simulink model "Trigonometry"  (R2017b)
settings: Solver=FixedStepAuto  StartTime=0.0  StopTime=10.0  FixedStep=0.1  RelTol=1e-3  EnableMultiTasking=on
model workspace (MAT data in the model file):
  lustrec_slx_eps = 0.001
settings Model: Creator=ktrinh  LastModifiedBy=hbourbou
settings DataIOCC: SaveFormat=StructureWithTime
settings OptimizationCC: LifeSpan=inf
settings DebuggingCC: SFUnexpectedBacktrackingDiag=warning  SFNoUnconditionalDefaultTransitionDiag=warning  SFExecutionAtInitializationDiag=none
settings HardwareCC: ProdBitPerSizeT=32  ProdBitPerPtrDiffT=32  ProdWordSize=32  ProdHWDeviceType=Specified
settings CodeAppCC: StateflowObjectComments=on
settings GRTTargetCC: TargetLangStandard=C89/C90 (ANSI)  GeneratePreprocessorConditionals=Disable all
settings ConfigComp: CovMetricSettings=dw  CovHtmlReporting=on  CovSaveCumulativeToWorkspaceVar=on  CovSaveSingleToWorkspaceVar=on  CovExternalEMLEnable=off

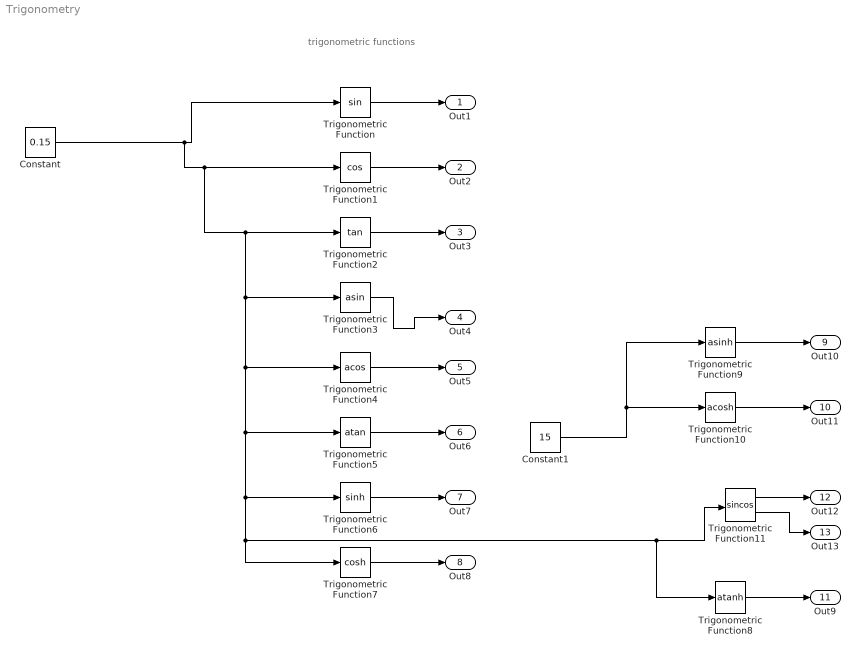
== system Trigonometry ==
  note: trigonometric functions
  Constant : Constant  Value=0.15
  Constant1 : Constant  Value=15
  Trigonometric Function : Trigonometry  ApproximationMethod=CORDIC
  Trigonometric Function1 : Trigonometry  Operator=cos  ApproximationMethod=CORDIC
  Trigonometric Function10 : Trigonometry  Operator=acosh  ApproximationMethod=CORDIC
  Trigonometric Function11 : Trigonometry  Operator=sincos  ApproximationMethod=CORDIC
  Trigonometric Function2 : Trigonometry  Operator=tan  ApproximationMethod=CORDIC
  Trigonometric Function3 : Trigonometry  Operator=asin  ApproximationMethod=CORDIC
  Trigonometric Function4 : Trigonometry  Operator=acos  ApproximationMethod=CORDIC
  Trigonometric Function5 : Trigonometry  Operator=atan  ApproximationMethod=CORDIC
  Trigonometric Function6 : Trigonometry  Operator=sinh  ApproximationMethod=CORDIC
  Trigonometric Function7 : Trigonometry  Operator=cosh  ApproximationMethod=CORDIC
  Trigonometric Function8 : Trigonometry  Operator=atanh  ApproximationMethod=CORDIC
  Trigonometric Function9 : Trigonometry  Operator=asinh  ApproximationMethod=CORDIC
  Out1 : Outport
  Out2 : Outport  Port=2
  Out3 : Outport  Port=3
  Out4 : Outport  Port=4
  Out5 : Outport  Port=5
  Out6 : Outport  Port=6
  Out7 : Outport  Port=7
  Out8 : Outport  Port=8
  Out10 : Outport  Port=9
  Out11 : Outport  Port=10
  Out9 : Outport  Port=11
  Out12 : Outport  Port=12
  Out13 : Outport  Port=13
  wires:
  Trigonometric Function/1 -> Out1/1
  Trigonometric Function1/1 -> Out2/1
  Trigonometric Function2/1 -> Out3/1
  Trigonometric Function3/1 -> Out4/1
  Trigonometric Function4/1 -> Out5/1
  Trigonometric Function5/1 -> Out6/1
  Trigonometric Function6/1 -> Out7/1
  Trigonometric Function7/1 -> Out8/1
  Trigonometric Function9/1 -> Out10/1
  Trigonometric Function10/1 -> Out11/1
  Constant/1 -> Trigonometric Function8/1, Trigonometric Function11/1, Trigonometric Function7/1, Trigonometric Function6/1, Trigonometric Function5/1, Trigonometric Function4/1, Trigonometric Function3/1, Trigonometric Function2/1, Trigonometric Function1/1, Trigonometric Function/1
  Trigonometric Function8/1 -> Out9/1
  Trigonometric Function11/1 -> Out12/1
  Trigonometric Function11/2 -> Out13/1
  Constant1/1 -> Trigonometric Function10/1, Trigonometric Function9/1
